simulink model "Ex4Lista3"  (R2022b)
settings: Solver=VariableStepAuto  StartTime=0.0  StopTime=10  RelTol=1e-3
settings Model: Creator=vfton  LastModifiedBy=matak
settings DebuggingCC: AlgebraicLoopMsg=none
settings ModelReferenceCC: EnableRefExpFcnMdlSchedulingChecks=on

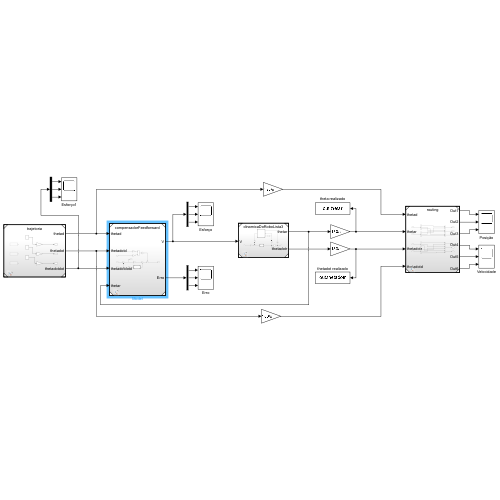
[thumbnail: Simulink's stored preview of the top-level diagram]
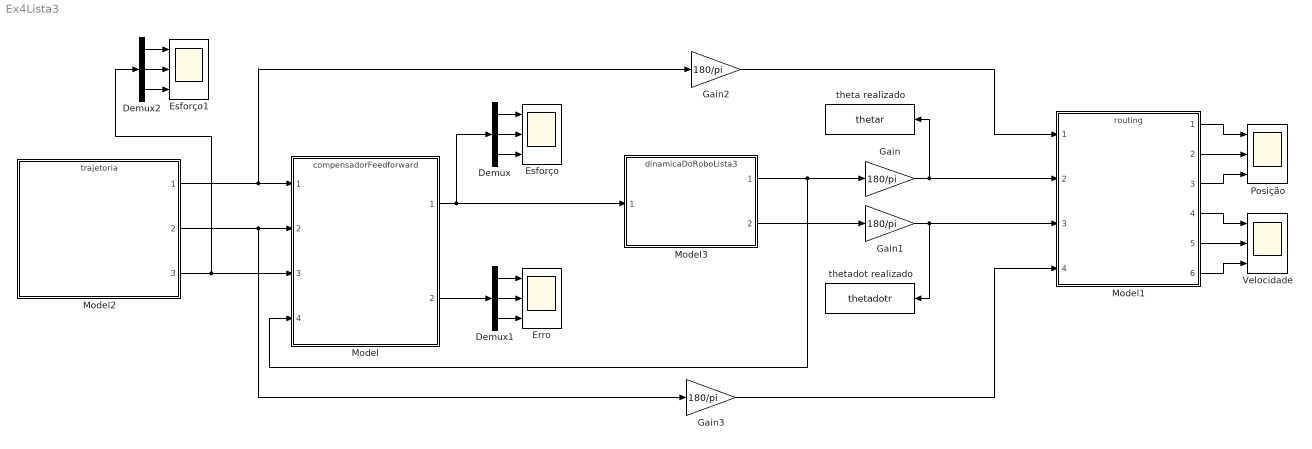
== system Ex4Lista3 ==
  Demux : Demux  Outputs=3
  Demux1 : Demux  Outputs=3
  Demux2 : Demux  Outputs=3
  Erro : Scope  NumInputPorts=3
  Esforço : Scope  NumInputPorts=3
  Esforço1 : Scope  NumInputPorts=3
  Gain{,1..3} (4 alike) : Gain  Gain=180/pi
  Model : ModelReference  ModelNameDialog=compensadorFeedforward.slx  SimulationMode=Normal  ModelReferenceVersion=1.6
  Model1 : ModelReference  ModelNameDialog=routing.slx  SimulationMode=Normal  ModelReferenceVersion=1.1
  Model2 : ModelReference  ModelNameDialog=trajetoria.slx  SimulationMode=Normal  ModelReferenceVersion=2.0
  Model3 : ModelReference  ModelNameDialog=dinamicaDoRoboLista3.slx  SimulationMode=Normal  ModelReferenceVersion=1.7
  Posição : Scope  NumInputPorts=3
  Velocidade : Scope  NumInputPorts=3
  theta realizado : ToWorkspace  VariableName=thetar  SaveFormat=Timeseries  SampleTime=-1
  thetadot realizado : ToWorkspace  VariableName=thetadotr  SaveFormat=Timeseries  SampleTime=-1
  wires:
  Model/1 -> Model3/1, Demux/1
  Demux/2 -> Esforço/2
  Demux/1 -> Esforço/1
  Demux/3 -> Esforço/3
  Demux1/1 -> Erro/1
  Demux1/2 -> Erro/2
  Demux1/3 -> Erro/3
  Model/2 -> Demux1/1
  Model3/1 -> Model/4, Gain/1
  Model3/2 -> Gain1/1
  Gain/1 -> Model1/2, theta realizado/1
  Gain1/1 -> thetadot realizado/1, Model1/3
  Model2/2 -> Gain3/1, Model/2
  Model1/2 -> Posição/2
  Model1/1 -> Posição/1
  Model1/3 -> Posição/3
  Model1/4 -> Velocidade/1
  Model1/5 -> Velocidade/2
  Model1/6 -> Velocidade/3
  Model2/3 -> Demux2/1, Model/3
  Model2/1 -> Gain2/1, Model/1
  Demux2/3 -> Esforço1/3
  Demux2/1 -> Esforço1/1
  Demux2/2 -> Esforço1/2
  Gain2/1 -> Model1/1
  Gain3/1 -> Model1/4
